simulink model "ModeS_Simulink_libiio_org"  (Simulink 10.0)
settings: Solver=VariableStepDiscrete  StartTime=0.0  StopTime=3e6  RelTol=1e-3
PreLoadFcn:
  | load data_Yb
  | DataIn = Yb_with_time(:,2);
  | WL=14;
  | n = length(DataIn);
undefined symbols (not defined in the file): dfilt
libraries: simulink_need_slupdate x24, simulink x3, dspobslib x2, commutil2 x1, hdlsllib x1, dspindex x1, dspbuff3 x1, dspsrcs4 x1
settings Model: Creator=mdonovan  LastModifiedBy=annonymous
settings DataIOCC: LimitDataPoints=on  SignalLoggingSaveFormat=ModelDataLogs  SaveOutput=off  SignalLogging=off  SaveTime=off
settings OptimizationCC: BlockReduction=off  BooleanDataType=off  ConditionallyExecuteInputs=off  DefaultParameterBehavior=Inlined  ExpressionDepthLimit=2147483647  LocalBlockOutputs=off
settings DebuggingCC: AlgebraicLoopMsg=error  SolverPrmCheckMsg=warning  SingleTaskRateTransMsg=error  FcnCallInpInsideContextMsg=warning  StateNameClashWarn=warning
settings GRTTargetCC: GeneratePreprocessorConditionals=Disable all
settings ConfigComp: CovExternalEMLEnable=off  CovSFcnEnable=off

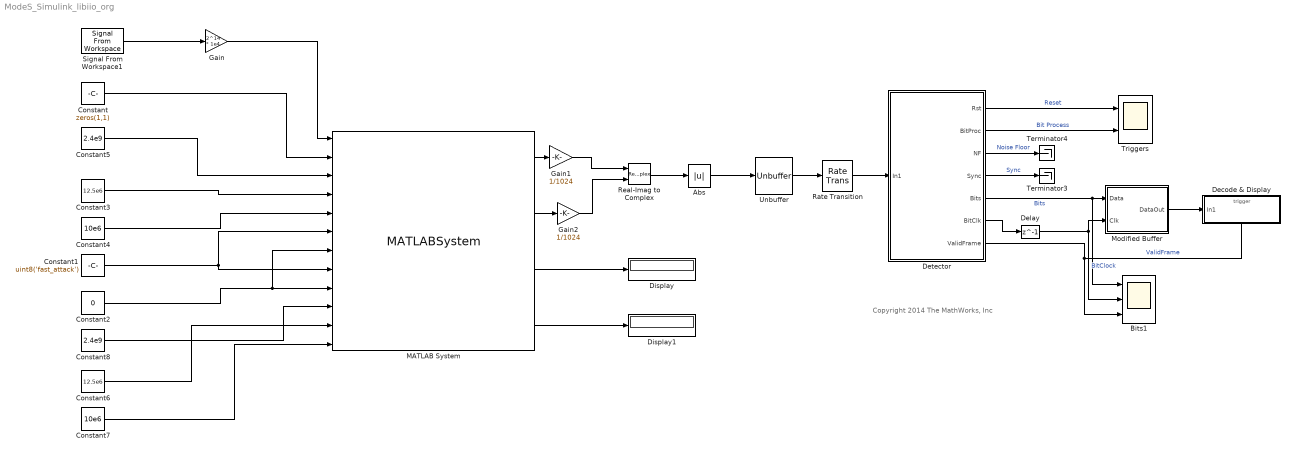
== system ModeS_Simulink_libiio_org ==
  note: Copyright 2014 The MathWorks, Inc
  Abs : Abs
  Bits1 : Scope  NumInputPorts=3
  Constant : Constant  Value=zeros(1,1)  VectorParams1D=off  FramePeriod=1e6
      settings: SamplingMode=Frame based
  Constant1 : Constant  Value=uint8('fast_attack')  SampleTime=-1
  Constant2 : Constant  Value=0  SampleTime=-1
  Constant3 : Constant  Value=12.5e6  SampleTime=-1
  Constant4 : Constant  Value=10e6  SampleTime=-1
  Constant5 : Constant  Value=2.4e9  SampleTime=-1
  Constant6 : Constant  Value=12.5e6  SampleTime=-1
  Constant7 : Constant  Value=10e6  SampleTime=-1
  Constant8 : Constant  Value=2.4e9  SampleTime=-1
  Decode & Display : Subsystem
  Delay : Delay  DelayLength=1
  Detector : Subsystem
  Display : Display
  Display1 : Display
  Gain : Gain  Gain=2^14 * 1e4
  Gain1 : Gain  Gain=1/1024
  Gain2 : Gain  Gain=1/1024
  MATLAB System : MATLABSystem  DialogController=sysobjdialog.BlockDynDialog  System=iio_sys_obj  ip_address=192.168.3.2  dev_name=ad9361  in_ch_no=2  in_ch_size=1e6  out_ch_no=2  out_ch_size=1e6  SimulateUsing=Interpreted execution
      mask Type: iio_sys_obj
      mask Display:
      | disp('ad9361');
      | port_label('input',1,'DATA_IN1');
      | port_label('input',2,'DATA_IN2');
      | port_label('input',3,'RX_LO_FREQ');
      | port_label('input',4,'RX_SAMPLING_FREQ');
      | port_label('input',5,'RX_RF_BANDWIDTH');
      | port_label('input',6,'RX1_GAIN_MODE');
      | port_label('input',7,'RX1_GAIN');
      | port_label('input',8,'RX2_GAIN_MODE');
      | port_label('input',9,'RX2_GAIN');
      | port_label('input',10,'TX_LO_FREQ');
      | port_label('input',11,'TX_SAMPLING_FREQ');
      | port_label('input',12,'TX_RF_BANDWIDTH');
      | port_label('output',1,'DATA_OUT1');
      | port_label('output',2,'DATA_OUT2');
      | port_label('output',3,'RX1_RSSI');
      | port_label('output',4,'RX2_RSSI');
  Modified Buffer : Subsystem  TreatAsAtomicUnit=on  mask(Input-Driven Buffer){bufSize=112}
      mask prompts: bufSize "Buffer size:"
      mask help: A modified buffer subsystem that is driven by the arrival of its input data; it produces a valid output data buffer whenever its buffer is full and sets its dataValid flag to 1. Otherwise, the data at its dataOut port is not valid and its dataValid flag is set to 0.
  Rate Transition : RateTransition
  Real-Imag to Complex : RealImagToComplex
  Signal From Workspace1 : dspsrcs4/Signal From Workspace  X=DataIn  Ts=1  nsamps=1e6  OutputAfterFinalValue=Cyclic repetition  ignoreOrWarnInputAndFrameLengths=off  OutputFrames=on
  Terminator3 : Terminator
  Terminator4 : Terminator
  Triggers : Scope  NumInputPorts=2
  Unbuffer : Unbuffer
  wires:
  MATLAB System/1 -> Gain1/1
  Signal From Workspace1/1 -> Gain/1
  Constant/1 -> MATLAB System/2
  MATLAB System/2 -> Gain2/1
  Detector/5(Bits) -> Bits1/1, Modified Buffer/1(Data)  "Bits"
  Modified Buffer/1(DataOut) -> Decode & Display/1(In1)
  Delay/1 -> Bits1/2, Modified Buffer/2(Clk)  "BitClock"
  Detector/6(BitClk) -> Delay/1
  Detector/7(ValidFrame) -> Decode & Display/Trigger, Bits1/3  "ValidFrame"
  Detector/3(NF) -> Terminator4/1  "Noise Floor"
  Detector/4(Sync) -> Terminator3/1  "Sync"
  Detector/1(Rst) -> Triggers/1  "Reset"
  Detector/2(BitProc) -> Triggers/2  "Bit Process"
  MATLAB System/3 -> Display/1
  MATLAB System/4 -> Display1/1
  Constant5/1 -> MATLAB System/3
  Constant3/1 -> MATLAB System/4
  Constant4/1 -> MATLAB System/5
  Constant6/1 -> MATLAB System/11
  Constant7/1 -> MATLAB System/12
  Constant1/1 -> MATLAB System/8, MATLAB System/6
  Constant2/1 -> MATLAB System/7, MATLAB System/9
  Constant8/1 -> MATLAB System/10
  Unbuffer/1 -> Rate Transition/1
  Rate Transition/1 -> Detector/1(In1)
  Gain/1 -> MATLAB System/1
  Real-Imag to Complex/1 -> Abs/1
  Gain1/1 -> Real-Imag to Complex/1
  Gain2/1 -> Real-Imag to Complex/2
  Abs/1 -> Unbuffer/1

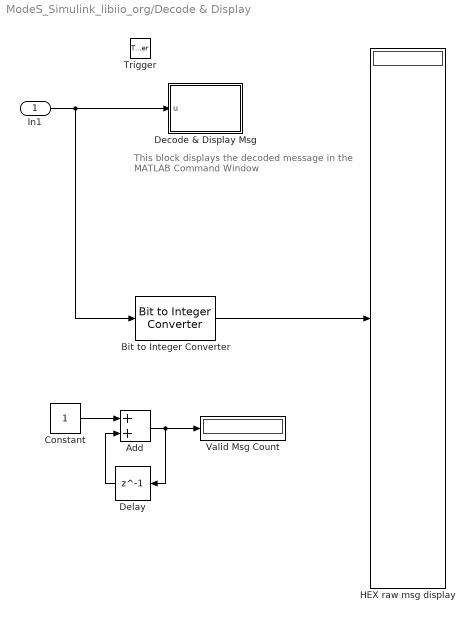
== system ModeS_Simulink_libiio_org/Decode & Display ==
  note: This block displays the decoded message in
      | the MATLAB Command Window
  In1 : Inport
  Trigger : TriggerPort  VariantControl=Variant
  Add : Sum
  Bit to Integer Converter : commutil2/Bit to Integer Converter  nbits=4  bitOrder=MSB first  signedOutputValues=Unsigned  outDtype=Inherit via internal rule  outDtypeSigned=Inherit via internal rule
      settings: SourceProductName=Communications Toolbox
  Constant : Constant
  Decode & Display Msg : MATLAB Function  TreatAsAtomicUnit=on
  Delay : Delay  DelayLength=1
  HEX raw msg display : Display
      settings: Format=hex (Stored Integer)
  Valid Msg Count : Display
  wires:
  In1/1 -> Decode & Display Msg/1(u), Bit to Integer Converter/1
  Add/1 -> Valid Msg Count/1, Delay/1
  Constant/1 -> Add/1
  Delay/1 -> Add/2
  Bit to Integer Converter/1 -> HEX raw msg display/1

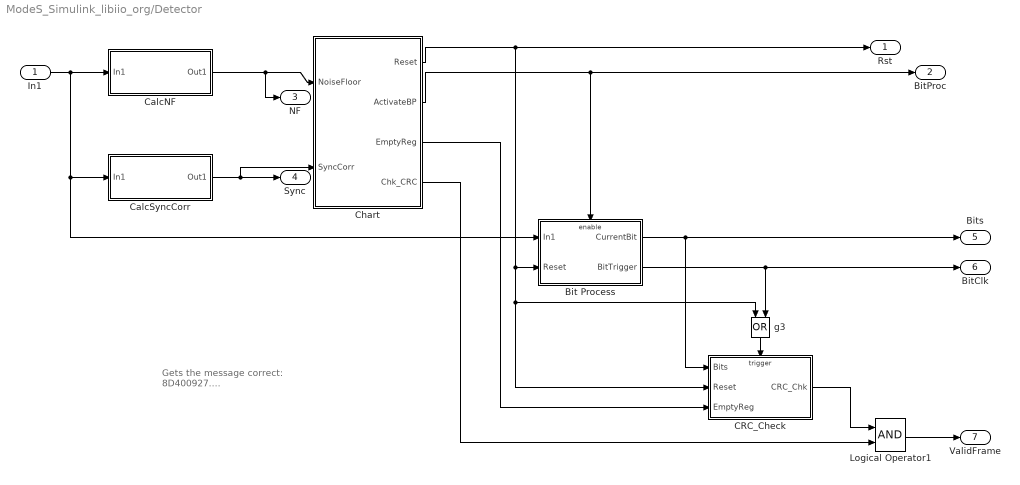
== system ModeS_Simulink_libiio_org/Detector ==
  note: Gets the message correct:
      | 8D400927....
  In1 : Inport
  Bit Process : Subsystem  TreatAsAtomicUnit=on
  CRC_Check : Subsystem
  CalcNF : Subsystem
  CalcSyncCorr : Subsystem
  Chart : Stateflow chart  TreatAsAtomicUnit=on
  Logical Operator1 : Logic  AllPortsSameDT=off  OutDataTypeStr=boolean
  g3 : Logic  Operator=OR  AllPortsSameDT=off  OutDataTypeStr=boolean
  Rst : Outport
  BitProc : Outport  Port=2
  NF : Outport  Port=3
  Sync : Outport  Port=4
  Bits : Outport  Port=5
  BitClk : Outport  Port=6
  ValidFrame : Outport  Port=7
  wires:
  Chart/1(Reset) -> Rst/1, Bit Process/2(Reset), CRC_Check/2(Reset), g3/1
  Bit Process/1(CurrentBit) -> CRC_Check/1(Bits), Bits/1
  Chart/3(EmptyReg) -> CRC_Check/3(EmptyReg)
  Chart/2(ActivateBP) -> BitProc/1, Bit Process/Enable
  Bit Process/2(BitTrigger) -> g3/2, BitClk/1
  g3/1 -> CRC_Check/Trigger
  In1/1 -> CalcNF/1(In1), CalcSyncCorr/1(In1), Bit Process/1(In1)
  CalcNF/1(Out1) -> Chart/1(NoiseFloor), NF/1
  CalcSyncCorr/1(Out1) -> Sync/1, Chart/2(SyncCorr)
  Logical Operator1/1 -> ValidFrame/1
  CRC_Check/1(CRC_Chk) -> Logical Operator1/1
  Chart/4(Chk_CRC) -> Logical Operator1/2

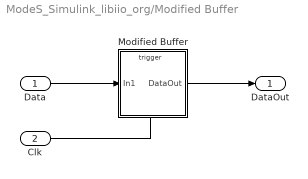
== system ModeS_Simulink_libiio_org/Modified Buffer ==
  Data : Inport
  Clk : Inport  Port=2
  Modified Buffer : Subsystem
  DataOut : Outport
  wires:
  Modified Buffer/1(DataOut) -> DataOut/1
  Clk/1 -> Modified Buffer/Trigger
  Data/1 -> Modified Buffer/1(In1)

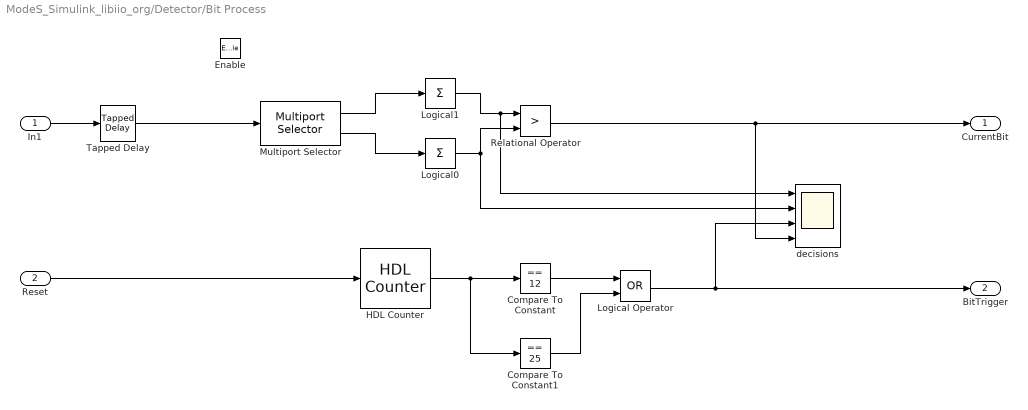
== system ModeS_Simulink_libiio_org/Detector/Bit Process ==
  In1 : Inport
  Reset : Inport  Port=2
  Enable : EnablePort
  Compare To Constant : simulink/Logic and Bit Operations/Compare To Constant  relop===  const=12  OutDataTypeStr=boolean
  Compare To Constant1 : simulink/Logic and Bit Operations/Compare To Constant  relop===  const=25  OutDataTypeStr=boolean
  HDL Counter : hdlsllib/HDL Operations/HDL Counter  CountType=Count limited  CountInit=1  CountStep=1  CountMax=25  CountFromType=Initial value  CountFrom=1  CountResetPort=on  CountLoadPort=off  CountEnbPort=off  CountDirPort=off  CountDataType=Unsigned  CountWordLen=8  CountFracLen=0  CountSampTime=1
      settings: SourceProductName=Simulink  SourceProductBaseCode=SL
  Logical Operator : Logic  Operator=OR  AllPortsSameDT=off  OutDataTypeStr=boolean
  Logical0 : Sum  Inputs=+  AccumDataTypeStr=double  OutDataTypeStr=Inherit: Same as accumulator
  Logical1 : Sum  Inputs=+  AccumDataTypeStr=double  OutDataTypeStr=Inherit: Same as accumulator
  Multiport Selector : dspindex/Multiport Selector  rowsOrCols=Rows  idxCellArray={ 1:6,7:12}  idxErrMode=Clip Index
  Relational Operator : RelationalOperator  Operator=>  OutDataTypeStr=boolean  RndMeth=Nearest
  Tapped Delay : simulink/Discrete/Tapped Delay  vinit=0.0  samptime=1  NumDelays=12  DelayOrder=Oldest  includeCurrent=on
  decisions : Scope  NumInputPorts=4
  CurrentBit : Outport  InitialOutput=0
  BitTrigger : Outport  Port=2  InitialOutput=0
  wires:
  Tapped Delay/1 -> Multiport Selector/1
  Multiport Selector/1 -> Logical1/1
  Multiport Selector/2 -> Logical0/1
  Logical1/1 -> Relational Operator/1, decisions/1
  Logical0/1 -> Relational Operator/2, decisions/2
  In1/1 -> Tapped Delay/1
  Reset/1 -> HDL Counter/1
  HDL Counter/1 -> Compare To Constant/1, Compare To Constant1/1
  Compare To Constant/1 -> Logical Operator/1
  Compare To Constant1/1 -> Logical Operator/2
  Relational Operator/1 -> CurrentBit/1, decisions/4
  Logical Operator/1 -> BitTrigger/1, decisions/3

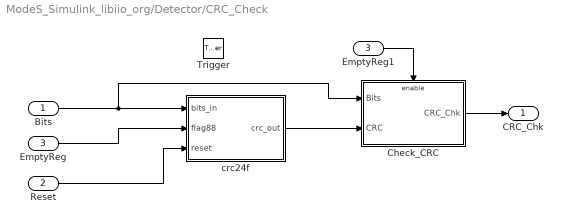
== system ModeS_Simulink_libiio_org/Detector/CRC_Check ==
  Bits : Inport
  Reset : Inport  Port=2
  EmptyReg : Inport  Port=3
  Trigger : TriggerPort  VariantControl=Variant
  Check_CRC : Subsystem  TreatAsAtomicUnit=on
  EmptyReg1 : InportShadow  Port=3
  crc24f : Subsystem
  CRC_Chk : Outport
  wires:
  Bits/1 -> crc24f/1(bits_in), Check_CRC/1(Bits)
  EmptyReg/1 -> crc24f/2(flag88)
  Reset/1 -> crc24f/3(reset)
  crc24f/1(crc_out) -> Check_CRC/2(CRC)
  EmptyReg1/1 -> Check_CRC/Enable
  Check_CRC/1(CRC_Chk) -> CRC_Chk/1

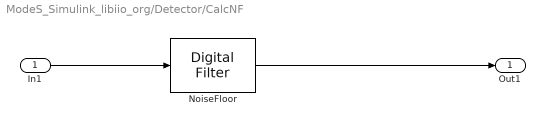
== system ModeS_Simulink_libiio_org/Detector/CalcNF ==
  In1 : Inport
  NoiseFloor : dspobslib/Digital Filter  TypePopup=FIR (all zeros)  IIRFiltStruct=Direct form II transposed  AllPoleFiltStruct=Direct form  FIRFiltStruct=Direct form transposed  CoeffSource=Specify via dialog  NumCoeffs=(ones(64,1)/64)  DenCoeffs=[1 0.1]  BiQuadCoeffs=[1 0.3 0.4 1 0.1 0.2]  LatticeCoeffs=[0.2 0.4]  denIgnore=on  FiltPerSampPopup=One filter per frame  IC=0  ICnum=0  ICden=0  firstCoeffMode=Binary point scaling  firstCoeffWordLength=WL  firstCoeffFracLength=WL + 4  outputMode=Binary point scaling  outputWordLength=WL  outputFracLength=WL + 8  accumMode=Binary point scaling  accumWordLength=2*WL  accumFracLength=2*WL + 8  prodOutputMode=Binary point scaling  prodOutputWordLength=2*WL  prodOutputFracLength=2*WL + 14  roundingMode=Floor  overflowMode=off  ScaleValues=1  scaleValueFracLength=14  stageInFracLength=15  stageOutFracLength=15  FilterSource=Specify via dialog  dfiltObjectName=dfilt.dffir([1 2 1])  InputProcessing=Columns as channels (frame based)
      settings: SourceProductName=DSP System Toolbox  SourceProductBaseCode=DS
  Out1 : Outport
  wires:
  In1/1 -> NoiseFloor/1
  NoiseFloor/1 -> Out1/1

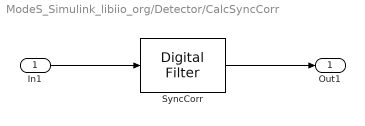
== system ModeS_Simulink_libiio_org/Detector/CalcSyncCorr ==
  In1 : Inport
  SyncCorr : dspobslib/Digital Filter  TypePopup=FIR (all zeros)  IIRFiltStruct=Direct form II transposed  AllPoleFiltStruct=Direct form  FIRFiltStruct=Direct form  CoeffSource=Specify via dialog  NumCoeffs=|  DenCoeffs=[1 0.1]  BiQuadCoeffs=[1 0.3 0.4 1 0.1 0.2]  LatticeCoeffs=[0.2 0.4]  denIgnore=on  FiltPerSampPopup=One filter per frame  IC=0  ICnum=0  ICden=0  firstCoeffMode=Binary point scaling  firstCoeffWordLength=WL  firstCoeffFracLength=WL - 2  outputMode=Binary point scaling  outputWordLength=WL  outputFracLength=WL + 4  accumMode=Binary point scaling  accumWordLength=2*WL  accumFracLength=2*WL + 4  prodOutputMode=Binary point scaling  prodOutputWordLength=2*WL  prodOutputFracLength=2*WL + 8  roundingMode=Floor  overflowMode=off  ScaleValues=1  scaleValueFracLength=14  stageInFracLength=15  stageOutFracLength=15  FilterSource=Specify via dialog  dfiltObjectName=dfilt.dffir([1 2 1])  InputProcessing=Columns as channels (frame based)
      | flipud([ones(6,1);-1*ones(6,1);ones(6,1);-1*ones(7,1);
      | -1*ones(6,1);-1*ones(6,1);-1*ones(6,1);ones(7,1);-1*ones(6,1);ones(6,1);-1*ones(6,1);-1*ones(7,1)])
      settings: SourceProductName=DSP System Toolbox  SourceProductBaseCode=DS
  Out1 : Outport
  wires:
  In1/1 -> SyncCorr/1
  SyncCorr/1 -> Out1/1

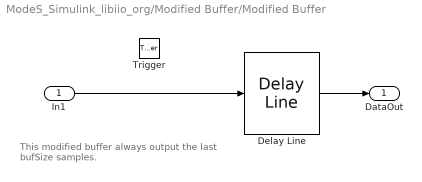
== system ModeS_Simulink_libiio_org/Modified Buffer/Modified Buffer ==
  note: This modified buffer always output the last
      | bufSize samples.
  In1 : Inport
  Trigger : TriggerPort  VariantControl=Variant
  Delay Line : dspbuff3/Delay Line  siz=bufSize  ic=0  directfeed=on  enable_output=off  hold_output=off  TreatMby1Signals=One channel  OutputFrames=on
      settings: SourceProductName=DSP System Toolbox  SourceProductBaseCode=DS
  DataOut : Outport
  wires:
  In1/1 -> Delay Line/1
  Delay Line/1 -> DataOut/1

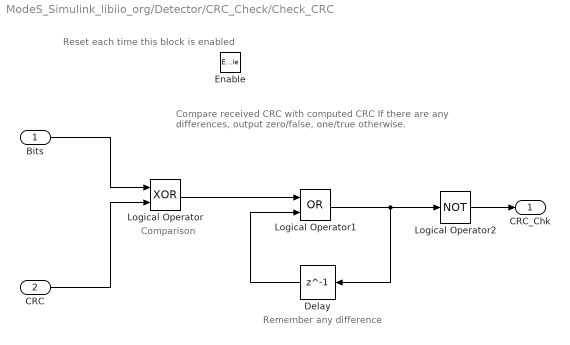
== system ModeS_Simulink_libiio_org/Detector/CRC_Check/Check_CRC ==
  note: Compare received CRC with computed CRC
      | If there are any differences, output zero/false, one/true otherwise.
  note: Comparison
  note: Remember any difference
  note: Reset each time this block is enabled
  Bits : Inport
  CRC : Inport  Port=2
  Enable : EnablePort  StatesWhenEnabling=reset
  Delay : Delay  DelayLength=1
  Logical Operator : Logic  Operator=XOR  AllPortsSameDT=off  OutDataTypeStr=boolean
  Logical Operator1 : Logic  Operator=OR  AllPortsSameDT=off  OutDataTypeStr=boolean
  Logical Operator2 : Logic  Operator=NOT  AllPortsSameDT=off  OutDataTypeStr=boolean
  CRC_Chk : Outport  InitialOutput=0
  wires:
  Bits/1 -> Logical Operator/1
  CRC/1 -> Logical Operator/2
  Logical Operator/1 -> Logical Operator1/1
  Delay/1 -> Logical Operator1/2
  Logical Operator1/1 -> Delay/1, Logical Operator2/1
  Logical Operator2/1 -> CRC_Chk/1

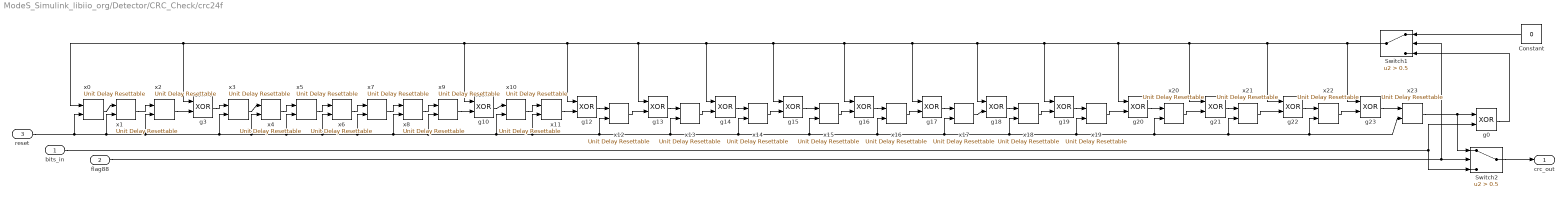
== system ModeS_Simulink_libiio_org/Detector/CRC_Check/crc24f ==
  bits_in : Inport
  flag88 : Inport  Port=2
  reset : Inport  Port=3
  Constant : Constant  Value=0  OutDataTypeStr=boolean  SampleTime=-1
  Switch1 : Switch  Criteria=u2 > Threshold  Threshold=0.5
  Switch2 : Switch  Criteria=u2 > Threshold  Threshold=0.5
  g{0,3,10,12..23} (15 alike) : Logic  Operator=XOR  AllPortsSameDT=off  OutDataTypeStr=boolean
  x{0..23} (24 alike) : simulink_need_slupdate/Unit Delay Resettable  vinit=0.0  tsamp=-1
      settings: SourceProductName=Simulink  SourceProductBaseCode=SL
  crc_out : Outport
  wires:
  x0/1 -> x1/1
  x1/1 -> x2/1
  x3/1 -> x4/1
  x4/1 -> x5/1
  x5/1 -> x6/1
  x6/1 -> x7/1
  x7/1 -> x8/1
  x8/1 -> x9/1
  x10/1 -> x11/1
  g3/1 -> x3/1
  x2/1 -> g3/2
  g10/1 -> x10/1
  x9/1 -> g10/2
  x11/1 -> g12/2
  g12/1 -> x12/1
  x12/1 -> g13/2
  g13/1 -> x13/1
  x13/1 -> g14/2
  g14/1 -> x14/1
  x14/1 -> g15/2
  g15/1 -> x15/1
  x15/1 -> g16/2
  g16/1 -> x16/1
  x16/1 -> g17/2
  g17/1 -> x17/1
  x17/1 -> g18/2
  g18/1 -> x18/1
  x18/1 -> g19/2
  g19/1 -> x19/1
  x19/1 -> g20/2
  g20/1 -> x20/1
  x20/1 -> g21/2
  g21/1 -> x21/1
  x21/1 -> g22/2
  g22/1 -> x22/1
  x22/1 -> g23/2
  g23/1 -> x23/1
  bits_in/1 -> g0/2, Switch2/3
  flag88/1 -> Switch2/2, Switch1/2
  x23/1 -> g0/1, Switch2/1
  Switch1/1 -> g10/1, g3/1, x0/1, g12/1, g13/1, g14/1, g15/1, g16/1, g17/1, g18/1, g19/1, g20/1, g21/1, g22/1, g23/1
  reset/1 -> x0/2, x1/2, x2/2, x3/2, x4/2, x5/2, x6/2, x7/2, x8/2, x9/2, x10/2, x11/2, x12/2, x13/2, x14/2, x15/2, x16/2, x17/2, x18/2, x19/2, x20/2, x21/2, x22/2, x23/2
  Constant/1 -> Switch1/1
  g0/1 -> Switch1/3
  Switch2/1 -> crc_out/1

== stateflow chart Detector/Chart ==
  settings: executeAtInitialization=1
  state SyncSearch
  state WaitForT0
    entry: T0Delay++;
  state BitProcess
    entry: SamplesIn++;
    Reset = 0;
  state ClearBP
    entry: SamplesIn++;
  state EmptyReg
    entry: CRCClocks++;
  (default) -> SyncSearch
  ClearBP -> SyncSearch [order 1] : [SamplesIn>100]
      | {Chk_CRC = 0;}
  SyncSearch -> WaitForT0 : [SyncCorr > 10*NoiseFloor]
      | {ActivateBP = 1;
      | maxSync = SyncCorr;
      | SamplesIn = 0;
      | T0Delay = 0;
      | Reset = 1;
      | Chk_CRC = 0;}
  WaitForT0 -> WaitForT0 [order 3]
  BitProcess -> WaitForT0 [order 2] : [SyncCorr > maxSync && SamplesIn < 50]
      | {Reset = 1;
      | SamplesIn = 0;
      | maxSync = SyncCorr;
      | T0Delay = 0;}
  WaitForT0 -> WaitForT0 [order 2] : [SyncCorr > maxSync]
      | {T0Delay = 0;
      | maxSync = SyncCorr;}
  WaitForT0 -> BitProcess [order 1] : [T0Delay>25]
  BitProcess -> BitProcess [order 3]
  ClearBP -> ClearBP [order 2] : {Chk_CRC = 0;}
  BitProcess -> EmptyReg [order 1] : [SamplesIn>=12.5*88]
      | {EmptyReg = 1;
      | CRCClocks = 0;}
  EmptyReg -> ClearBP [order 1] : [CRCClocks>=24*12.5]
      | {maxSync = 0;
      | ActivateBP = 0;
      | Reset = 0;
      | SamplesIn = 0;
      | EmptyReg = 0;
      | Chk_CRC = 1;}
  EmptyReg -> EmptyReg [order 2]
  data: NoiseFloor input double; SyncCorr input double; Reset output boolean =0; ActivateBP output boolean =0; EmptyReg output boolean =0; SamplesIn local uint16 =0; CRCClocks local uint16 =0; Chk_CRC output boolean =0; T0Delay local double; maxSync local double

== matlab function Decode & Display/Decode & Display Msg ==
  data: u input double
function MsgDecode(u)
%#codegen
coder.extrinsic('DecodeBits')
DecodeBits(single(u));

%d = bin2dec(num2str(c'));
% rxBytes = dec2hex(d)';
